simulink model "clutch_lock_up_model"  (R2020b)
settings: Solver=VariableStepAuto  StartTime=0.0  StopTime=10.0  RelTol=1e-3
model workspace (MAT data in the model file):
  input_torque_data = Simulink.SimulationData.Dataset
  input_torque_data.any.Name = ''
  input_torque_data.any.Version = 3
  input_torque_data.any.Storage = Simulink.SimulationData.Storage.RamDatasetStorage
  input_torque_data.any.Storage.any.Version = 2
  input_torque_data.any.Storage.any.Elements{1} = Simulink.SimulationData.Signal
  input_torque_data.any.Storage.any.Elements{1}.Version = 1
  input_torque_data.any.Storage.any.Elements{1}.Values = timeseries
  input_torque_data.any.Storage.any.Elements{1}.Values.Name = 'unnamed'
  input_torque_data.any.Storage.any.Elements{1}.Values.DataInfo = tsdata.datametadata
  input_torque_data.any.Storage.any.Elements{1}.Values.DataInfo.Interpolation = tsdata.interpolation
  input_torque_data.any.Storage.any.Elements{1}.Values.DataInfo.Interpolation.Fhandle : function handle (value not decoded)
  input_torque_data.any.Storage.any.Elements{1}.Values.DataInfo.Interpolation.Name = 'linear'
  input_torque_data.any.Storage.any.Elements{1}.Values.TimeInfo = tsdata.timemetadata
  input_torque_data.any.Storage.any.Elements{1}.Values.TimeInfo.Length = 11
  input_torque_data.any.Storage.any.Elements{1}.Values.TimeInfo.DuplicateTimes = 0
  input_torque_data.any.Storage.any.Elements{1}.Values.TimeInfo.Time_ = [0; 1; 2; 3; 4; 5; 6; 7; 8; 9; 10]
  input_torque_data.any.Storage.any.Elements{1}.Values.TimeInfo.Initialized = 1
  input_torque_data.any.Storage.any.Elements{1}.Values.QualityInfo = tsdata.qualmetadata
  input_torque_data.any.Storage.any.Elements{1}.Values.Data_ = [2; 2; 2; 2; 2; 2; 0; 0; 0; 0; 0]
  input_torque_data.any.Storage.any.Elements{1}.Name = 'Ti'
  input_torque_dataCopy = Simulink.SimulationData.Dataset
  input_torque_dataCopy.any.Name = ''
  input_torque_dataCopy.any.Version = 3
  input_torque_dataCopy.any.Storage = Simulink.SimulationData.Storage.RamDatasetStorage
  input_torque_dataCopy.any.Storage.any.Version = 2
  input_torque_dataCopy.any.Storage.any.Elements{1} = Simulink.SimulationData.Signal
  input_torque_dataCopy.any.Storage.any.Elements{1}.Version = 1
  input_torque_dataCopy.any.Storage.any.Elements{1}.Values = timeseries
  input_torque_dataCopy.any.Storage.any.Elements{1}.Values.Name = 'unnamed'
  input_torque_dataCopy.any.Storage.any.Elements{1}.Values.DataInfo = tsdata.datametadata
  input_torque_dataCopy.any.Storage.any.Elements{1}.Values.DataInfo.Interpolation = tsdata.interpolation
  input_torque_dataCopy.any.Storage.any.Elements{1}.Values.DataInfo.Interpolation.Fhandle : function handle (value not decoded)
  input_torque_dataCopy.any.Storage.any.Elements{1}.Values.DataInfo.Interpolation.Name = 'linear'
  input_torque_dataCopy.any.Storage.any.Elements{1}.Values.TimeInfo = tsdata.timemetadata
  input_torque_dataCopy.any.Storage.any.Elements{1}.Values.TimeInfo.Length = 11
  input_torque_dataCopy.any.Storage.any.Elements{1}.Values.TimeInfo.DuplicateTimes = 0
  input_torque_dataCopy.any.Storage.any.Elements{1}.Values.TimeInfo.Time_ = [0; 1; 2; 3; 4; 5; 6; 7; 8; 9; 10]
  input_torque_dataCopy.any.Storage.any.Elements{1}.Values.TimeInfo.Initialized = 1
  input_torque_dataCopy.any.Storage.any.Elements{1}.Values.QualityInfo = tsdata.qualmetadata
  input_torque_dataCopy.any.Storage.any.Elements{1}.Values.Data_ = [2; 2; 2; 2; 2; 2; 0; 0; 0; 0; 0]
  input_torque_dataCopy.any.Storage.any.Elements{1}.Name = 'Ti'
  simin = [0  0; 1  0.8; 2  1.6; 3  1.6; 4  1.6; 5  1.6; 6  0.8; 7  0; 8  0; 9  0; 10  0]
values from neighbouring files (symbols this model uses):
  Be = 2.0    [model_parameters_of_clutch.sldd]
  Bv = 1.0    [model_parameters_of_clutch.sldd]
  Ie = 1.0    [model_parameters_of_clutch.sldd]
  Iv = 5.0    [model_parameters_of_clutch.sldd]
  R = 1.0    [model_parameters_of_clutch.sldd]
  uk = 1.0    [model_parameters_of_clutch.sldd]
  us = 1.5    [model_parameters_of_clutch.sldd]
settings Model: DataDictionary=model_parameters_of_clutch.sldd  OrderedModelArguments=off  Creator=153  LastModifiedBy=153
settings DataIOCC: ExternalInput="[Ti  Fn]"

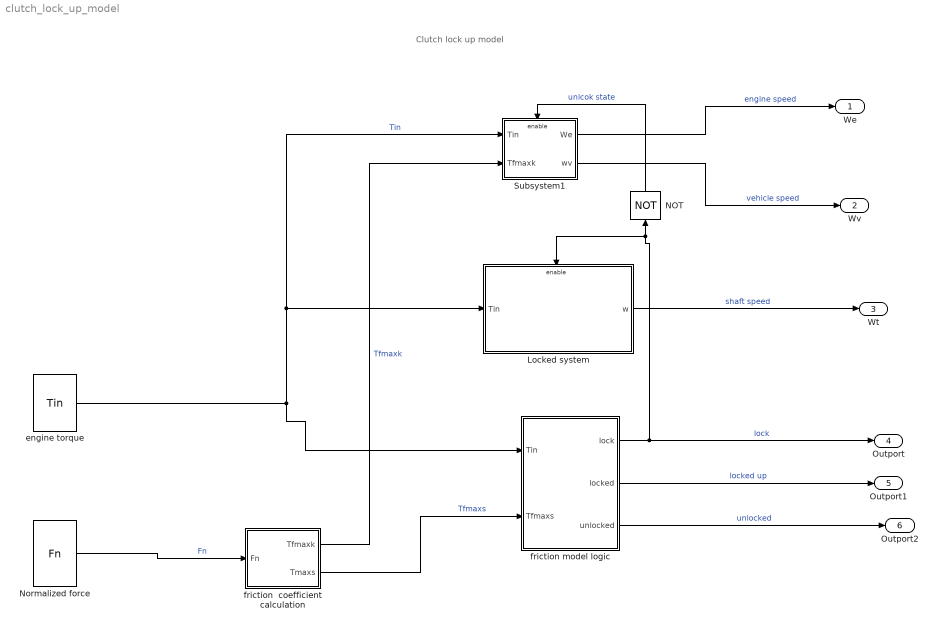
== system clutch_lock_up_model ==
  note: Clutch lock up model
  Locked system : Subsystem
  NOT : Logic  Operator=NOT  IconShape=distinctive  AllPortsSameDT=off  OutDataTypeStr=boolean
  Normalized force : FromWorkspace  VariableName=Fn
  Subsystem1 : Subsystem
  engine torque : FromWorkspace  VariableName=Tin
  friction  coefficient calculation : Subsystem
  friction model logic : Subsystem
  We : Outport
  Wv : Outport  Port=2
  Wt : Outport  Port=3
  Outport : Outport  Port=4
  Outport1 : Outport  Port=5
  Outport2 : Outport  Port=6
  wires:
  Normalized force/1 -> friction  coefficient calculation/1(Fn)  "Fn"
  engine torque/1 -> friction model logic/1(Tin), Subsystem1/1(Tin), Locked system/1(Tin)  "Tin"
  friction  coefficient calculation/2(Tmaxs) -> friction model logic/2(Tfmaxs)  "Tfmaxs"
  friction model logic/1(lock) -> Locked system/Enable, NOT/1, Outport/1  "lock"
  friction model logic/2(locked) -> Outport1/1  "locked up"
  friction model logic/3(unlocked) -> Outport2/1  "unlocked"
  Locked system/1(w) -> Wt/1  "shaft speed"
  friction  coefficient calculation/1(Tfmaxk) -> Subsystem1/2(Tfmaxk)  "Tfmaxk"
  Subsystem1/1(We) -> We/1  "engine speed"
  Subsystem1/2(wv) -> Wv/1  "vehicle speed"
  NOT/1 -> Subsystem1/Enable  "unlcok state"

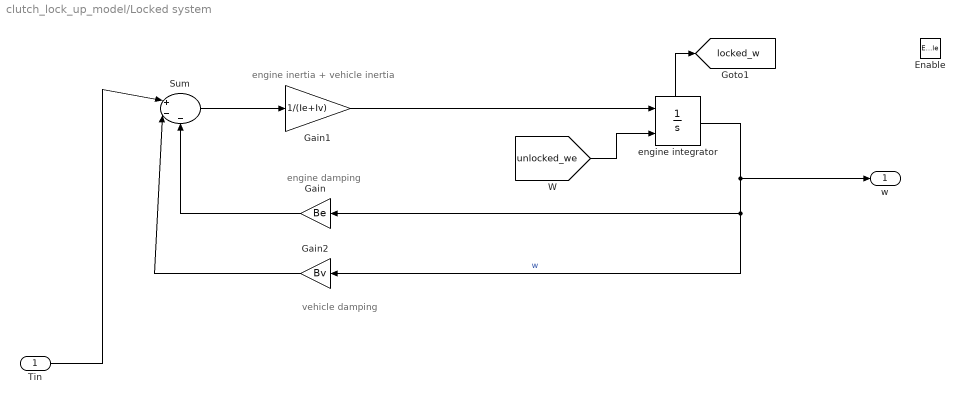
== system clutch_lock_up_model/Locked system ==
  note: engine damping
  note: engine inertia + vehicle inertia
  note: vehicle damping
  Tin : Inport
  Enable : EnablePort
  Gain : Gain  Gain=Be
  Gain1 : Gain  Gain=1/(Ie+Iv)
  Gain2 : Gain  Gain=Bv
  Sum : Sum  Inputs=|+--
  engine integrator : Integrator  InitialConditionSource=external  ShowStatePort=on
  w : Outport
  tag scope: locked_w=global
  wires:
  Sum/1 -> Gain1/1
  Tin/1 -> Sum/1
  engine integrator/1 -> w/1, Gain/1, Gain2/1  "w"
  engine integrator/State -> [locked_w]
  Gain2/1 -> Sum/2
  Gain/1 -> Sum/3
  Gain1/1 -> engine integrator/1
  [unlocked_we] -> engine integrator/2

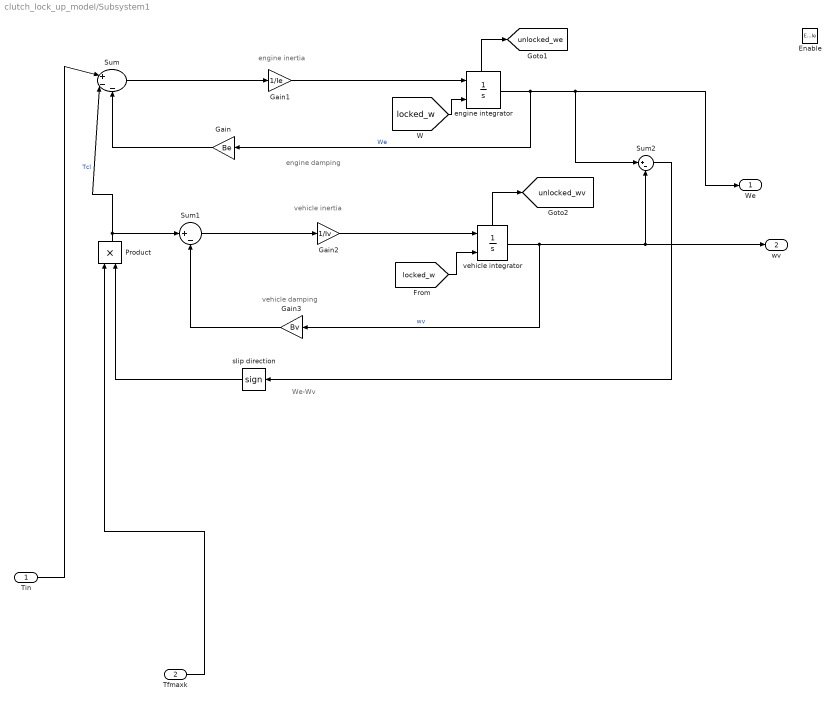
== system clutch_lock_up_model/Subsystem1 ==
  note: engine inertia
  note: engine damping
  note: vehicle inertia
  note: vehicle damping
  note: We-Wv
  Tin : Inport
  Tfmaxk : Inport  Port=2
  Enable : EnablePort
  Gain : Gain  Gain=Be
  Gain1 : Gain  Gain=1/Ie
  Gain2 : Gain  Gain=1/Iv
  Gain3 : Gain  Gain=Bv
  Product : Product
  Sum : Sum  Inputs=|+--
  Sum1 : Sum  Inputs=|+-
  Sum2 : Sum  Inputs=|+-
  engine integrator : Integrator  InitialConditionSource=external  ShowStatePort=on
  slip direction : Signum
  vehicle integrator : Integrator  InitialConditionSource=external  ShowStatePort=on
  We : Outport
  wv : Outport  Port=2
  tag scope: unlocked_we=global, unlocked_wv=global
  wires:
  engine integrator/State -> [unlocked_we]
  Sum2/1 -> slip direction/1
  Sum1/1 -> Gain2/1
  Gain1/1 -> engine integrator/1
  Gain/1 -> Sum/3
  slip direction/1 -> Product/2
  vehicle integrator/State -> [unlocked_wv]
  [locked_w] -> vehicle integrator/2
  Sum/1 -> Gain1/1
  Gain3/1 -> Sum1/2
  vehicle integrator/1 -> wv/1, Sum2/2, Gain3/1  "wv"
  engine integrator/1 -> We/1, Sum2/1, Gain/1  "We"
  Product/1 -> Sum/2, Sum1/1  "Tcl"
  Gain2/1 -> vehicle integrator/1
  [locked_w] -> engine integrator/2
  Tfmaxk/1 -> Product/1
  Tin/1 -> Sum/1

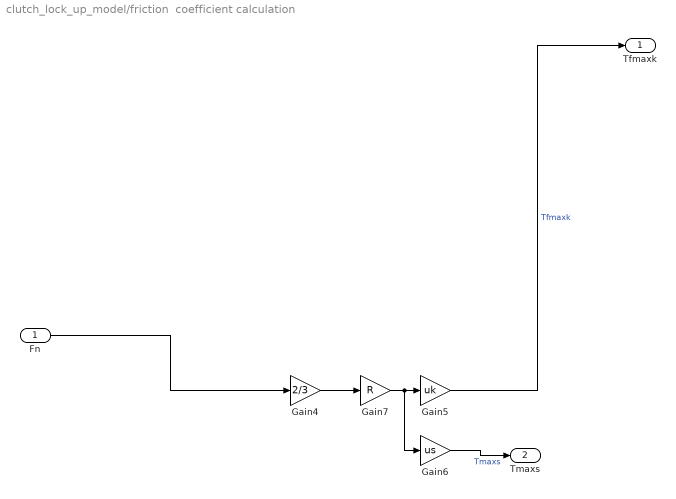
== system clutch_lock_up_model/friction  coefficient calculation ==
  Fn : Inport
  Gain4 : Gain  Gain=2/3
  Gain5 : Gain  Gain=uk
  Gain6 : Gain  Gain=us
  Gain7 : Gain  Gain=R
  Tfmaxk : Outport
  Tmaxs : Outport  Port=2
  wires:
  Gain7/1 -> Gain6/1, Gain5/1
  Gain4/1 -> Gain7/1
  Gain6/1 -> Tmaxs/1  "Tmaxs"
  Gain5/1 -> Tfmaxk/1  "Tfmaxk"
  Fn/1 -> Gain4/1

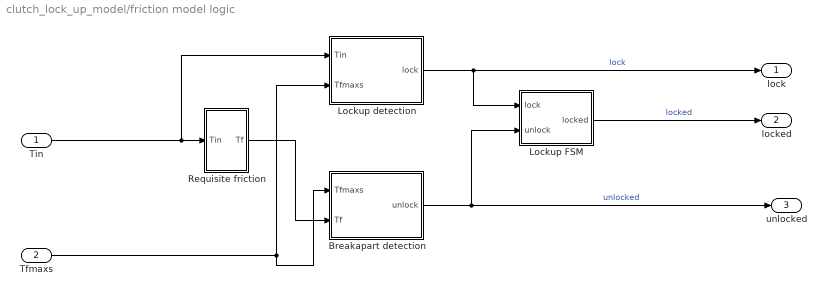
== system clutch_lock_up_model/friction model logic ==
  Tin : Inport
  Tfmaxs : Inport  Port=2
  Breakapart detection : Subsystem
  Lockup FSM : Subsystem
  Lockup detection : Subsystem
  Requisite friction : Subsystem
  lock : Outport
  locked : Outport  Port=2
  unlocked : Outport  Port=3
  wires:
  Breakapart detection/1(unlock) -> unlocked/1, Lockup FSM/2(unlock)  "unlocked"
  Lockup detection/1(lock) -> lock/1, Lockup FSM/1(lock)  "lock"
  Tin/1 -> Lockup detection/1(Tin), Requisite friction/1(Tin)
  Requisite friction/1(Tf) -> Breakapart detection/2(Tf)
  Tfmaxs/1 -> Lockup detection/2(Tfmaxs), Breakapart detection/1(Tfmaxs)
  Lockup FSM/1(locked) -> locked/1  "locked"

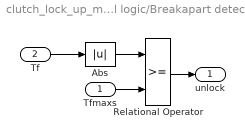
== system clutch_lock_up_model/friction model logic/Breakapart detection ==
  Tfmaxs : Inport
  Tf : Inport  Port=2
  Abs : Abs  SaturateOnIntegerOverflow=on
  Relational Operator : RelationalOperator  OutDataTypeStr=boolean  RndMeth=Nearest  InputSameDT=on
  unlock : Outport  InitialOutput=0  VectorParamsAs1DForOutWhenUnconnected=off
  wires:
  Tf/1 -> Abs/1
  Relational Operator/1 -> unlock/1
  Abs/1 -> Relational Operator/1
  Tfmaxs/1 -> Relational Operator/2

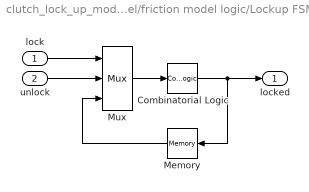
== system clutch_lock_up_model/friction model logic/Lockup FSM ==
  lock : Inport
  unlock : Inport  Port=2
  Combinatorial Logic : CombinatorialLogic  TruthTable=[0;1;0;0;1;1;1;0]
  Memory : Memory
  Mux : Mux  Inputs=3
  locked : Outport  InitialOutput=0  VectorParamsAs1DForOutWhenUnconnected=off
  wires:
  Memory/1 -> Mux/3
  Combinatorial Logic/1 -> locked/1, Memory/1
  unlock/1 -> Mux/2
  lock/1 -> Mux/1
  Mux/1 -> Combinatorial Logic/1

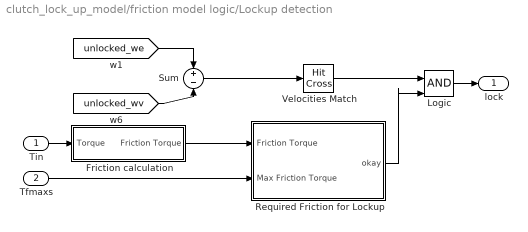
== system clutch_lock_up_model/friction model logic/Lockup detection ==
  Tin : Inport
  Tfmaxs : Inport  Port=2
  Friction calculation : Subsystem
  Logic : Logic  IconShape=distinctive  OutDataTypeStr=boolean
  Required Friction for Lockup : Subsystem
  Sum : Sum  Inputs=+-  InputSameDT=on  SaturateOnIntegerOverflow=on  OutDataTypeStr=Inherit: Same as first input
  Velocities Match : HitCross
  lock : Outport  InitialOutput=0  VectorParamsAs1DForOutWhenUnconnected=off
  wires:
  Friction calculation/1(Friction Torque) -> Required Friction for Lockup/1(Friction Torque)
  Tfmaxs/1 -> Required Friction for Lockup/2(Max Friction Torque)
  Velocities Match/1 -> Logic/1
  Logic/1 -> lock/1
  Required Friction for Lockup/1(okay) -> Logic/2
  [unlocked_we] -> Sum/1
  [unlocked_wv] -> Sum/2
  Sum/1 -> Velocities Match/1
  Tin/1 -> Friction calculation/1(Torque)

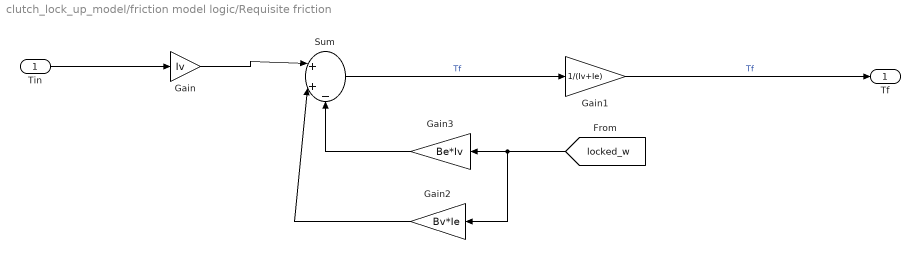
== system clutch_lock_up_model/friction model logic/Requisite friction ==
  Tin : Inport
  Gain : Gain  Gain=Iv
  Gain1 : Gain  Gain=1/(Iv+Ie)
  Gain2 : Gain  Gain=Bv*Ie
  Gain3 : Gain  Gain=Be*Iv
  Sum : Sum  Inputs=|++-
  Tf : Outport
  wires:
  Gain3/1 -> Sum/3
  Gain2/1 -> Sum/2
  Gain/1 -> Sum/1
  Tin/1 -> Gain/1
  Sum/1 -> Gain1/1  "Tf"
  Gain1/1 -> Tf/1  "Tf"
  [locked_w] -> Gain2/1, Gain3/1

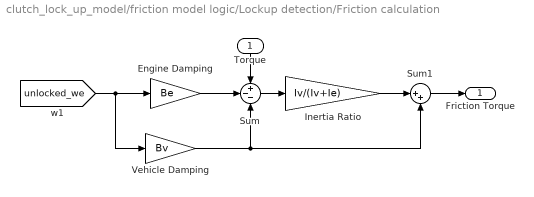
== system clutch_lock_up_model/friction model logic/Lockup detection/Friction calculation ==
  Torque : Inport
  Engine Damping : Gain  Gain=Be  SaturateOnIntegerOverflow=on  OutDataTypeStr=Inherit: Same as input  ParamDataTypeStr=Inherit: Same as input
  Inertia Ratio : Gain  Gain=Iv/(Iv+Ie)  SaturateOnIntegerOverflow=on  OutDataTypeStr=Inherit: Same as input  ParamDataTypeStr=Inherit: Same as input
  Sum : Sum  Inputs=+--  InputSameDT=on  SaturateOnIntegerOverflow=on  OutDataTypeStr=Inherit: Same as first input
  Sum1 : Sum  Inputs=|++  InputSameDT=on  SaturateOnIntegerOverflow=on  OutDataTypeStr=Inherit: Same as first input
  Vehicle Damping : Gain  Gain=Bv  SaturateOnIntegerOverflow=on  OutDataTypeStr=Inherit: Same as input  ParamDataTypeStr=Inherit: Same as input
  Friction Torque : Outport  InitialOutput=0  VectorParamsAs1DForOutWhenUnconnected=off
  wires:
  [unlocked_we] -> Engine Damping/1, Vehicle Damping/1
  Vehicle Damping/1 -> Sum1/2, Sum/3
  Engine Damping/1 -> Sum/2
  Sum/1 -> Inertia Ratio/1
  Torque/1 -> Sum/1
  Inertia Ratio/1 -> Sum1/1
  Sum1/1 -> Friction Torque/1

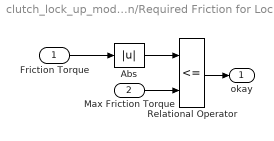
== system clutch_lock_up_model/friction model logic/Lockup detection/Required Friction for Lockup ==
  Friction Torque : Inport
  Max Friction Torque : Inport  Port=2
  Abs : Abs  SaturateOnIntegerOverflow=on
  Relational Operator : RelationalOperator  Operator=<=  OutDataTypeStr=boolean  RndMeth=Nearest  InputSameDT=on
  okay : Outport  InitialOutput=0  VectorParamsAs1DForOutWhenUnconnected=off
  wires:
  Friction Torque/1 -> Abs/1
  Relational Operator/1 -> okay/1
  Abs/1 -> Relational Operator/1
  Max Friction Torque/1 -> Relational Operator/2
